simulink model "BMS_EstimateSOC_COM_Harness_SIL"  (R2022b)
settings: configuration reference "BMS_Sw_CodeGenConfig" (kept outside this file)
undefined symbols (not defined in the file): BATT, DiscIntNeverNeededParam, Ion, Lithium, Schedule
libraries: simulink x4, spsIdealSwitchLib x3, pil_lib x1, spsBatteryLib x1, spsParallelRLCBranchLib x1, spspowerguiLib x1
settings Model: DataDictionary=BMS_Arch_DD.sldd  Creator=MAAM  LastModifiedBy=MAAM
settings ConfigSetRef: SourceName=BMS_Sw_CodeGenConfig

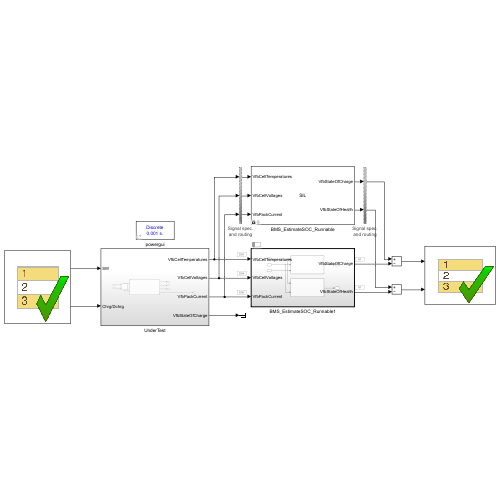
[thumbnail: Simulink's stored preview of the top-level diagram]
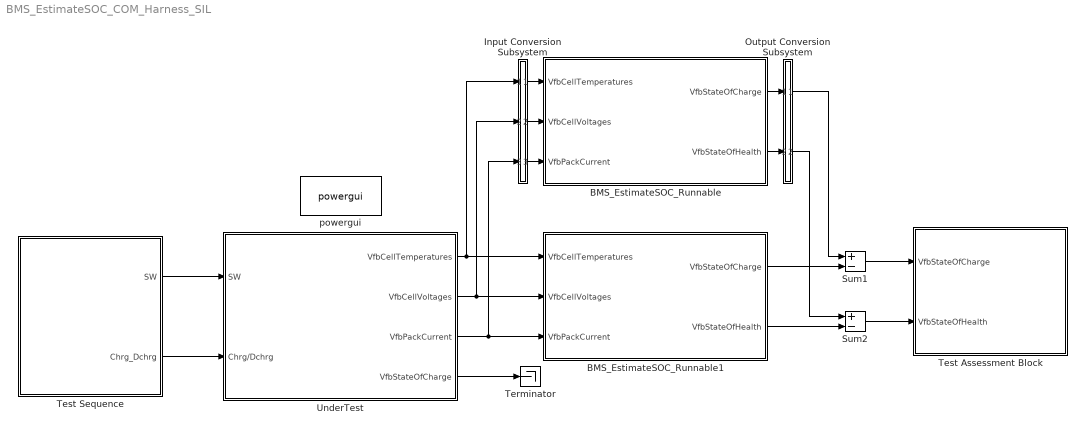
== system BMS_EstimateSOC_COM_Harness_SIL ==
  BMS_EstimateSOC_Runnable : Subsystem  Tag=__SL_testing_harness_stub_  DialogController=pil_create_dialog  LoadFcn=|
      | try
      |    if ~strcmp(rtw.pil.getPILVersion, '9.13 (R2022b)_15')
      |       set_param(gcb, 'DialogController', '');
      |       set_param(gcb, 'DialogControllerArgs', '');
      |    end
      | catch e
      |       set_param(gcb, 'DialogController', '');
      |       set_param(gcb, 'DialogControllerArgs', '');
      | end
      mask help: PIL:pil:XILBlockMaskDesc
      mask Display: disp('SIL');
  BMS_EstimateSOC_Runnable1 : Subsystem  Tag=BMS_EstimateSOC_Task  Priority=3  TreatAsAtomicUnit=on  ScheduleAs=Periodic partition  PartitionName=BMS_EstimateSOC_Task  SystemSampleTime=Schedule.BMS_EstimateSOC_Task
      settings: RTWSystemCode=Nonreusable function  RTWFcnNameOpts=Use subsystem name  FunctionInterfaceSpec=Allow arguments (Optimized)
  Input Conversion Subsystem : Subsystem  Tag=__SLT_ICS__  Description=|
      | Signal spec.
      | and routing
      settings: AttributesFormatString=%<Description>
  Output Conversion Subsystem : Subsystem  Tag=__SLT_OCS__  Description=|
      | Signal spec.
      | and routing
      settings: AttributesFormatString=%<Description>
  Sum1 : Sum  Inputs=+-
  Sum2 : Sum  Inputs=+-
  Terminator : Terminator
  Test Assessment Block : Test Sequence  Tag=__SLT_ASMT__  TreatAsAtomicUnit=on
  Test Sequence : Test Sequence  TreatAsAtomicUnit=on
  UnderTest : Subsystem
  powergui : spspowerguiLib/powergui  Priority=1  SimulationMode=Discrete  SampleTime=1e-3  frequency=60  Iterations=50  frequencyindice=0  Pbase=100e6  ErrMax=1e-4  UnitsV=kV  UnitsW=MW  buscounter=0  FunctionMessages=off  echomessages=off  EnableUseOfTLC=off  CurrentSourceSwitches=off  DisableSnubberDevices=off  DisableRonSwitches=off  DisableVfSwitches=off  DisplayEquations=off  AutomaticDiscreteSolvers=off  SolverType=Tustin/Backward Euler (TBE)  Interpol=off  ExternalGateDelay=off  methode=off  Ts=100  x0status=blocks  SPID=on  SwTol=0  HookPort=off  NonlinearTolerance=1e-4  nMaxIteration=100  ContinueOnMaxIteration=off  RestoreLinks=warning  ResistiveCurrentMeasurement=off  Frange=[0:2:500]  Ylog=off  Xlog=on  ShowGrid=off  save=off  variable=ZData  structure=0  ZoomFFT=off  StartTime=0.0  cycles=1  DisplayStyle=1  fundamental=60  FreqAxis=off  MaxFrequency=1000  frequencyindicesteady=1  RmsSteady=1  display=off
  wires:
  BMS_EstimateSOC_Runnable/1(VfbStateOfCharge) -> Output Conversion Subsystem/1(Inport_1)
  BMS_EstimateSOC_Runnable/2(VfbStateOfHealth) -> Output Conversion Subsystem/2(Inport_2)
  Input Conversion Subsystem/1(Outport_1) -> BMS_EstimateSOC_Runnable/1(VfbCellTemperatures)
  Input Conversion Subsystem/2(Outport_2) -> BMS_EstimateSOC_Runnable/2(VfbCellVoltages)
  Input Conversion Subsystem/3(Outport_3) -> BMS_EstimateSOC_Runnable/3(VfbPackCurrent)
  BMS_EstimateSOC_Runnable1/1(VfbStateOfCharge) -> Sum1/2
  BMS_EstimateSOC_Runnable1/2(VfbStateOfHealth) -> Sum2/2
  Test Sequence/1(SW) -> UnderTest/1(SW)
  Test Sequence/2(Chrg_Dchrg) -> UnderTest/2(Chrg/Dchrg)
  UnderTest/1(VfbCellTemperatures) -> Input Conversion Subsystem/1(Inport_1), BMS_EstimateSOC_Runnable1/1(VfbCellTemperatures)
  UnderTest/2(VfbCellVoltages) -> BMS_EstimateSOC_Runnable1/2(VfbCellVoltages), Input Conversion Subsystem/2(Inport_2)
  UnderTest/3(VfbPackCurrent) -> BMS_EstimateSOC_Runnable1/3(VfbPackCurrent), Input Conversion Subsystem/3(Inport_3)
  UnderTest/4(VfbStateOfCharge) -> Terminator/1
  Sum1/1 -> Test Assessment Block/1(VfbStateOfCharge)
  Sum2/1 -> Test Assessment Block/2(VfbStateOfHealth)
  Output Conversion Subsystem/2(Outport_2) -> Sum2/1
  Output Conversion Subsystem/1(Outport_1) -> Sum1/1

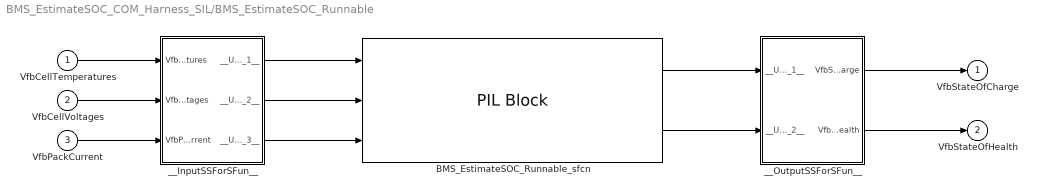
== system BMS_EstimateSOC_COM_Harness_SIL/BMS_EstimateSOC_Runnable ==
  VfbCellTemperatures : Inport  PortDimensions=BATT.Package.NumModules
  VfbCellVoltages : Inport  Port=2  PortDimensions=BATT.Package.NumModules
  VfbPackCurrent : Inport  Port=3
  BMS_EstimateSOC_Runnable_sfcn : pil_lib/PIL Block  SimulationMode=SIL  IsTopModelPIL=off  CodeDir=BMS_EstimateSOC_Runnable_ert_rtw  AnchorDir=H:\0\New MAAM\10 - MBD\Battary Management System  ConfigName=Software-in-the-Loop (SIL)  XrelIsTopModelCode=on  XrelIsReusable=off  XrelDWorkNames={}  XrelDWorkTypes={}  XrelModelArgVals={}  XrelOrderedParamNames={}
  __InputSSForSFun__ : Subsystem
  __OutputSSForSFun__ : Subsystem
  VfbStateOfCharge : Outport
  VfbStateOfHealth : Outport  Port=2
  wires:
  __OutputSSForSFun__/2(VfbStateOfHealth) -> VfbStateOfHealth/1
  __OutputSSForSFun__/1(VfbStateOfCharge) -> VfbStateOfCharge/1
  BMS_EstimateSOC_Runnable_sfcn/2 -> __OutputSSForSFun__/2(__UniqueInportName__2__)
  BMS_EstimateSOC_Runnable_sfcn/1 -> __OutputSSForSFun__/1(__UniqueInportName__1__)
  __InputSSForSFun__/3(__UniqueOutportName__3__) -> BMS_EstimateSOC_Runnable_sfcn/3
  __InputSSForSFun__/2(__UniqueOutportName__2__) -> BMS_EstimateSOC_Runnable_sfcn/2
  __InputSSForSFun__/1(__UniqueOutportName__1__) -> BMS_EstimateSOC_Runnable_sfcn/1
  VfbPackCurrent/1 -> __InputSSForSFun__/3(VfbPackCurrent)
  VfbCellVoltages/1 -> __InputSSForSFun__/2(VfbCellVoltages)
  VfbCellTemperatures/1 -> __InputSSForSFun__/1(VfbCellTemperatures)

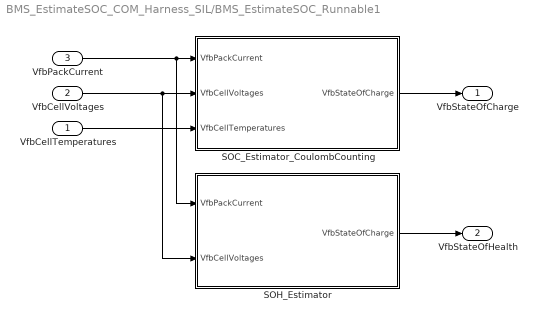
== system BMS_EstimateSOC_COM_Harness_SIL/BMS_EstimateSOC_Runnable1 ==
  VfbCellTemperatures : Inport  PortDimensions=BATT.Package.NumModules
  VfbCellVoltages : Inport  Port=2  PortDimensions=BATT.Package.NumModules
  VfbPackCurrent : Inport  Port=3
  SOC_Estimator_CoulombCounting : Subsystem  TreatAsAtomicUnit=on
      settings: RTWSystemCode=Nonreusable function  FunctionInterfaceSpec=Allow arguments (Optimized)
  SOH_Estimator : Subsystem  TreatAsAtomicUnit=on
      settings: RTWSystemCode=Nonreusable function  FunctionInterfaceSpec=Allow arguments (Optimized)
  VfbStateOfCharge : Outport
  VfbStateOfHealth : Outport  Port=2
  wires:
  SOH_Estimator/1(VfbStateOfCharge) -> VfbStateOfHealth/1
  SOC_Estimator_CoulombCounting/1(VfbStateOfCharge) -> VfbStateOfCharge/1
  VfbCellTemperatures/1 -> SOC_Estimator_CoulombCounting/3(VfbCellTemperatures)
  VfbCellVoltages/1 -> SOC_Estimator_CoulombCounting/2(VfbCellVoltages), SOH_Estimator/2(VfbCellVoltages)
  VfbPackCurrent/1 -> SOC_Estimator_CoulombCounting/1(VfbPackCurrent), SOH_Estimator/1(VfbPackCurrent)

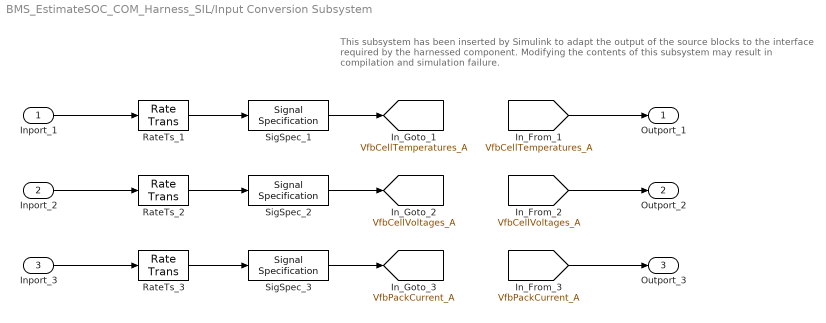
== system BMS_EstimateSOC_COM_Harness_SIL/Input Conversion Subsystem ==
  note: This subsystem has been inserted by Simulink to adapt the output of the source blocks to the interface required by the harnessed component.
      |  Modifying the contents of this subsystem may result in compilation and simulation failure.
  Inport_1 : Inport
  Inport_2 : Inport  Port=2
  Inport_3 : Inport  Port=3
  RateTs_1 : RateTransition  OutPortSampleTime=0.2
  RateTs_2 : RateTransition  OutPortSampleTime=0.2
  RateTs_3 : RateTransition  OutPortSampleTime=0.2
  SigSpec_1 : SignalSpecification  OutDataTypeStr=single  Unit=°C  Dimensions=[3]  SampleTime=0.2
  SigSpec_2 : SignalSpecification  OutDataTypeStr=single  Unit=V  Dimensions=[3]  SampleTime=0.2
  SigSpec_3 : SignalSpecification  OutDataTypeStr=single  Unit=A  Dimensions=[1]  SampleTime=0.2
  Outport_1 : Outport
  Outport_2 : Outport  Port=2
  Outport_3 : Outport  Port=3
  tag scope: VfbCellTemperatures_A=global, VfbCellVoltages_A=global, VfbPackCurrent_A=global
  wires:
  [VfbCellTemperatures_A] -> Outport_1/1
  SigSpec_1/1 -> [VfbCellTemperatures_A]
  RateTs_1/1 -> SigSpec_1/1
  Inport_1/1 -> RateTs_1/1
  [VfbCellVoltages_A] -> Outport_2/1
  SigSpec_2/1 -> [VfbCellVoltages_A]
  RateTs_2/1 -> SigSpec_2/1
  Inport_2/1 -> RateTs_2/1
  [VfbPackCurrent_A] -> Outport_3/1
  SigSpec_3/1 -> [VfbPackCurrent_A]
  RateTs_3/1 -> SigSpec_3/1
  Inport_3/1 -> RateTs_3/1

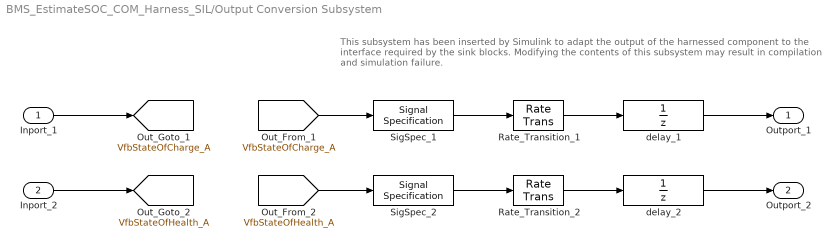
== system BMS_EstimateSOC_COM_Harness_SIL/Output Conversion Subsystem ==
  note: This subsystem has been inserted by Simulink to adapt the output of the harnessed component to the interface required by the sink blocks.
      |  Modifying the contents of this subsystem may result in compilation and simulation failure.
  Inport_1 : Inport
  Inport_2 : Inport  Port=2
  Rate_Transition_1 : RateTransition  OutPortSampleTimeOpt=Inherit
  Rate_Transition_2 : RateTransition  OutPortSampleTimeOpt=Inherit
  SigSpec_1 : SignalSpecification  OutDataTypeStr=single  Dimensions=[3]  SampleTime=0.2
  SigSpec_2 : SignalSpecification  OutDataTypeStr=single  Dimensions=[3]  SampleTime=0.2
  delay_1 : UnitDelay  SampleTime=-1
  delay_2 : UnitDelay  SampleTime=-1
  Outport_1 : Outport
  Outport_2 : Outport  Port=2
  tag scope: VfbStateOfCharge_A=global, VfbStateOfHealth_A=global
  wires:
  Inport_1/1 -> [VfbStateOfCharge_A]
  [VfbStateOfCharge_A] -> SigSpec_1/1
  SigSpec_1/1 -> Rate_Transition_1/1
  Rate_Transition_1/1 -> delay_1/1
  delay_1/1 -> Outport_1/1
  Inport_2/1 -> [VfbStateOfHealth_A]
  [VfbStateOfHealth_A] -> SigSpec_2/1
  SigSpec_2/1 -> Rate_Transition_2/1
  Rate_Transition_2/1 -> delay_2/1
  delay_2/1 -> Outport_2/1

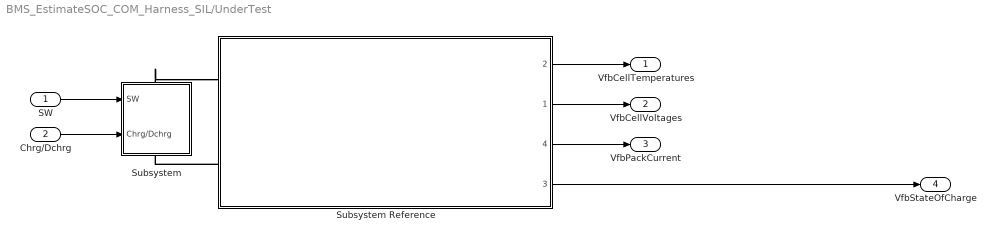
== system BMS_EstimateSOC_COM_Harness_SIL/UnderTest ==
  SW : Inport
  Chrg/Dchrg : Inport  Port=2
  Subsystem : Subsystem
      settings: PortSchema="{\"entries\":[{\"content\":{\"sides\":[{\"content\":{\"connectorIds\":[\"LConn1\"]},\"type\":\"ConnectorPlacement.EquallySpacedRectSide\",\"uuid\":\"a461fc5f-bdec-4de1-a769-19a6913359cb\"},{\"content\":{\"connectorIds\":[\"RConn1\"],\"side\":\"RIGHT\"},\"type\":\"ConnectorPlacement.EquallySpacedRectSide\",\"uuid\":\"53dfe770-afde-41f9-b1fd-6523bad3a9ef\"},{\"content\":{\"connectorIds\":[],\"side\":\"TOP\"},\"type\":\"ConnectorPlacement.EquallySpacedRectSide\",\"uuid\":\"157c2878-8b7f-49af-a18e-5ca91668c703\"},{\"content\":{\"connectorIds\":[\"In1\",\"In2\"],\"side\":\"BOTTOM\"},\"type\":\"ConnectorPlacement.EquallySpacedRectSide\",\"uuid\":\"a113e167-ab7e-4584-b97c-54a0a3809f54\"}]},\"type\":\"ConnectorPlacement.EquallySpacedConnector\",\"uuid\":\"fefc71e0-0cbe-4397-b099-f68d58411951\"}],\"packageUris\":[\"http://schema.mathworks.com/mf0/Connector/R2020b\"],\"version\":\"1.0\"}"
  Subsystem Reference : Subsystem  ReferencedSubsystem=Batter_Pack_Sim
      settings: PortSchema="{\"entries\":[{\"content\":{\"sides\":[{\"content\":{\"connectorIds\":[\"LConn1\",\"LConn2\"]},\"type\":\"ConnectorPlacement.EquallySpacedRectSide\",\"uuid\":\"5451cb71-15b5-4b08-b1e3-78543f6c5322\"},{\"content\":{\"connectorIds\":[\"Out2\",\"Out1\",\"Out4\",\"Out3\"],\"side\":\"RIGHT\"},\"type\":\"ConnectorPlacement.EquallySpacedRectSide\",\"uuid\":\"e4bd4e19-96bf-4958-bcea-cb5b9e999de9\"},{\"content\":{\"connectorIds\":[],\"side\":\"TOP\"},\"type\":\"ConnectorPlacement.EquallySpacedRectSide\",\"uuid\":\"ab10f796-18a4-45ff-a38a-380d34cf2a1b\"}]},\"type\":\"ConnectorPlacement.EquallySpacedConnector\",\"uuid\":\"eded12b9-95b7-465b-88e8-d172ae90f9f6\"}],\"packageUris\":[\"http://schema.mathworks.com/mf0/Connector/R2020b\"],\"version\":\"1.0\"}"
  VfbCellTemperatures : Outport
  VfbCellVoltages : Outport  Port=2
  VfbPackCurrent : Outport  Port=3
  VfbStateOfCharge : Outport  Port=4
  wires:
  Subsystem Reference/2 -> VfbCellTemperatures/1
  Subsystem Reference/1 -> VfbCellVoltages/1
  SW/1 -> Subsystem/1(SW)
  Subsystem Reference/3 -> VfbStateOfCharge/1
  Subsystem Reference/4 -> VfbPackCurrent/1
  Chrg/Dchrg/1 -> Subsystem/2(Chrg/Dchrg)
  connections:
  Subsystem/LConn1 -- Subsystem Reference/LConn1
  Subsystem Reference/LConn2 -- Subsystem/RConn1

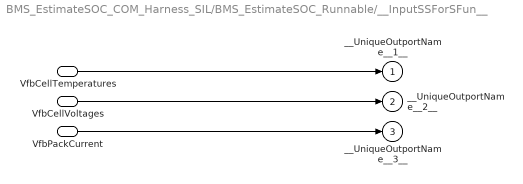
== system BMS_EstimateSOC_COM_Harness_SIL/BMS_EstimateSOC_Runnable/__InputSSForSFun__ ==
  VfbCellTemperatures : Inport  PortDimensions=BATT.Package.NumModules
  VfbCellVoltages : Inport  Port=2  PortDimensions=BATT.Package.NumModules
  VfbPackCurrent : Inport  Port=3
  __UniqueOutportName__1__ : Outport
  __UniqueOutportName__2__ : Outport  Port=2
  __UniqueOutportName__3__ : Outport  Port=3
  wires:
  VfbPackCurrent/1 -> __UniqueOutportName__3__/1
  VfbCellVoltages/1 -> __UniqueOutportName__2__/1
  VfbCellTemperatures/1 -> __UniqueOutportName__1__/1

== system BMS_EstimateSOC_COM_Harness_SIL/BMS_EstimateSOC_Runnable/__OutputSSForSFun__ ==
  __UniqueInportName__1__ : Inport
  __UniqueInportName__2__ : Inport  Port=2
  VfbStateOfCharge : Outport
  VfbStateOfHealth : Outport  Port=2
  wires:
  __UniqueInportName__2__/1 -> VfbStateOfHealth/1  "SOC"
  __UniqueInportName__1__/1 -> VfbStateOfCharge/1  "SOC"

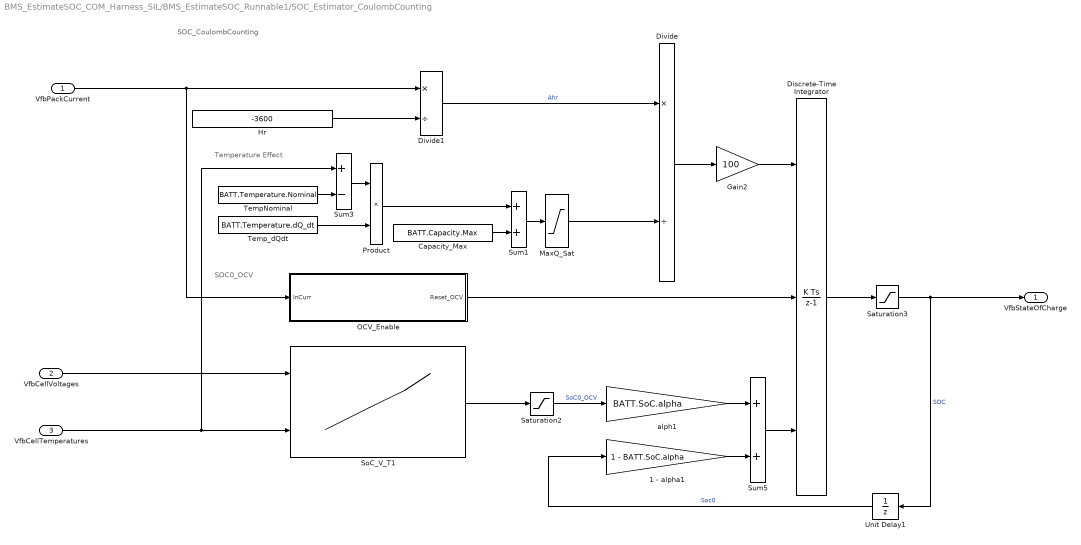
== system BMS_EstimateSOC_COM_Harness_SIL/BMS_EstimateSOC_Runnable1/SOC_Estimator_CoulombCounting ==
  note: SOC0_OCV
  note: Temperature Effect
  note: SOC_CoulombCounting
  VfbPackCurrent : Inport
  VfbCellVoltages : Inport  Port=2  PortDimensions=BATT.Package.NumModules
  VfbCellTemperatures : Inport  Port=3
  1 - alpha1 : Gain  Gain=1 - BATT.SoC.alpha
  Capacity_Max : Constant  Value=BATT.Capacity.Max
  Discrete-Time Integrator : DiscreteIntegrator  ExternalReset=rising  InitialConditionSource=external  InitialCondition=BATT.SOC.SoC0  SampleTime=-1  ICPrevOutput=DiscIntNeverNeededParam  ICPrevScaledInput=DiscIntNeverNeededParam
  Divide : Product  Inputs=*/  OutDataTypeStr=single
  Divide1 : Product  Inputs=*/
  Gain2 : Gain  Gain=100  OutDataTypeStr=single
  Hr : Constant  Value=-3600  OutDataTypeStr=single
  MaxQ_Sat : Saturate  UpperLimit=BATT.Capacity.Max  LowerLimit=0
  OCV_Enable : Subsystem
  Product : Product
  Saturation2 : Saturate  UpperLimit=BATT.SoC.max  LowerLimit=BATT.SoC.min  OutDataTypeStr=single
  Saturation3 : Saturate  UpperLimit=BATT.SoC.max  LowerLimit=BATT.SoC.min  OutDataTypeStr=single
  SoC_V_T1 : Lookup_n-D  BreakpointsForDimension1=BATT.Voltage.V_LUT  BreakpointsForDimension2=BATT.Temperature.T_LUT  Table=BATT.SoC.TableData  InternalRulePriority=Speed  RndMeth=Simplest
      settings: InputPortMap=u0,u1
  Sum1 : Sum
  Sum3 : Sum  Inputs=+-
  Sum5 : Sum
  TempNominal : Constant  Value=BATT.Temperature.Nominal
  Temp_dQdt : Constant  Value=BATT.Temperature.dQ_dt
  Unit Delay1 : UnitDelay  InitialCondition=BATT.SoC.SoC0 * ones(BATT.Package.Ns_Module, BATT.Package.NumModules)  SampleTime=-1  HasFrameUpgradeWarning=on
  alph1 : Gain  Gain=BATT.SoC.alpha
  VfbStateOfCharge : Outport
  wires:
  VfbPackCurrent/1 -> OCV_Enable/1(InCurr), Divide1/1
  VfbCellTemperatures/1 -> Sum3/1, SoC_V_T1/2
  VfbCellVoltages/1 -> SoC_V_T1/1
  Saturation3/1 -> VfbStateOfCharge/1, Unit Delay1/1  "SOC"
  TempNominal/1 -> Sum3/2
  Sum3/1 -> Product/1
  Temp_dQdt/1 -> Product/2
  Capacity_Max/1 -> Sum1/2
  Product/1 -> Sum1/1
  Sum1/1 -> MaxQ_Sat/1
  Divide1/1 -> Divide/1  "Ahr"
  Saturation2/1 -> alph1/1  "SoC0_OCV"
  Discrete-Time Integrator/1 -> Saturation3/1
  1 - alpha1/1 -> Sum5/2
  alph1/1 -> Sum5/1
  Divide/1 -> Gain2/1
  Sum5/1 -> Discrete-Time Integrator/3
  OCV_Enable/1(Reset_OCV) -> Discrete-Time Integrator/2
  Unit Delay1/1 -> 1 - alpha1/1  "Soc0"
  Gain2/1 -> Discrete-Time Integrator/1
  MaxQ_Sat/1 -> Divide/2
  Hr/1 -> Divide1/2
  SoC_V_T1/1 -> Saturation2/1

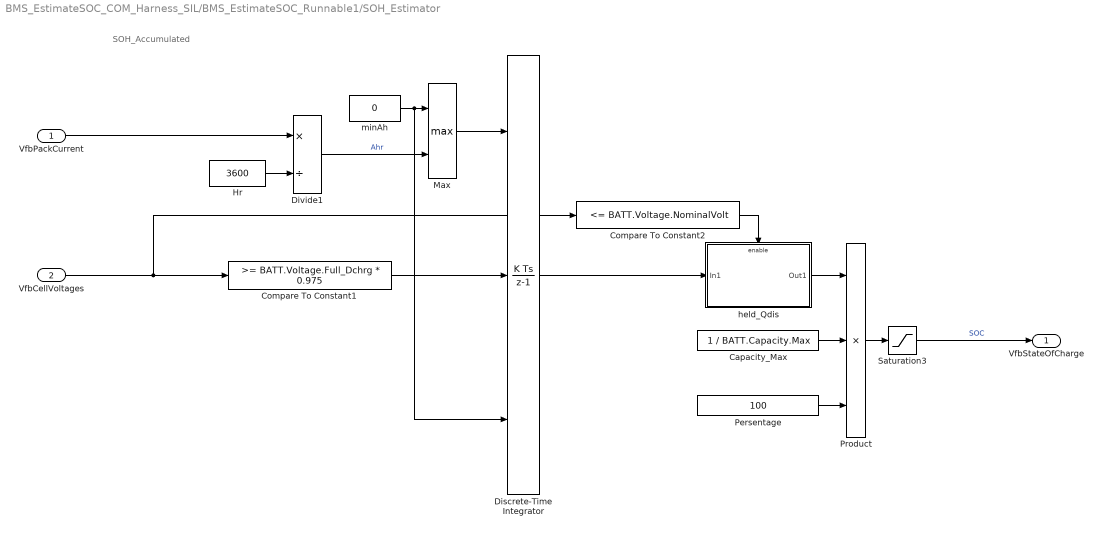
== system BMS_EstimateSOC_COM_Harness_SIL/BMS_EstimateSOC_Runnable1/SOH_Estimator ==
  note: SOH_Accumulated
  VfbPackCurrent : Inport
  VfbCellVoltages : Inport  Port=2  PortDimensions=BATT.Package.NumModules
  Capacity_Max : Constant  Value=1 / BATT.Capacity.Max
  Compare To Constant1 : simulink/Logic and Bit Operations/Compare To Constant  relop=>=  const=BATT.Voltage.Full_Dchrg * 0.975  OutDataTypeStr=boolean
  Compare To Constant2 : simulink/Logic and Bit Operations/Compare To Constant  relop=<=  const=BATT.Voltage.NominalVolt  OutDataTypeStr=boolean
  Discrete-Time Integrator : DiscreteIntegrator  ExternalReset=rising  InitialConditionSource=external  InitialCondition=BATT.SOC.SoC0  SampleTime=-1  ICPrevOutput=DiscIntNeverNeededParam  ICPrevScaledInput=DiscIntNeverNeededParam
  Divide1 : Product  Inputs=*/
  Hr : Constant  Value=3600  OutDataTypeStr=single
  Max : MinMax  Function=max  Inputs=2
  Persentage : Constant  Value=100
  Product : Product  Inputs=3
  Saturation3 : Saturate  UpperLimit=BATT.SoC.max  LowerLimit=BATT.SoC.min  OutDataTypeStr=single
  held_Qdis : Subsystem  TreatAsAtomicUnit=on
  minAh : Constant  Value=0  OutDataTypeStr=single
  VfbStateOfCharge : Outport
  wires:
  Persentage/1 -> Product/3
  Capacity_Max/1 -> Product/2
  held_Qdis/1(Out1) -> Product/1
  Compare To Constant2/1 -> held_Qdis/Enable
  Product/1 -> Saturation3/1
  Compare To Constant1/1 -> Discrete-Time Integrator/2
  Max/1 -> Discrete-Time Integrator/1
  minAh/1 -> Max/1, Discrete-Time Integrator/3
  Hr/1 -> Divide1/2
  Discrete-Time Integrator/1 -> held_Qdis/1(In1)
  Divide1/1 -> Max/2  "Ahr"
  Saturation3/1 -> VfbStateOfCharge/1  "SOC"
  VfbCellVoltages/1 -> Compare To Constant1/1, Compare To Constant2/1
  VfbPackCurrent/1 -> Divide1/1

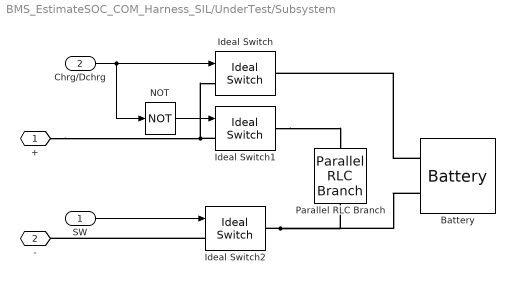
== system BMS_EstimateSOC_COM_Harness_SIL/UnderTest/Subsystem ==
  SW : Inport
  Chrg/Dchrg : Inport  Port=2
  Battery : spsBatteryLib/Battery  BatType=Lithium-Ion  ShowTempParam=off  ThermalPreset=no  ShowAgeParam=off  NomV=3*4.2  NomQ=150  SOC=100  Batt_Tr=1  PresetModel=on  MaxQ=150  MinV=9.45  FullV=14.6662  Dis_rate=65.2174  R=0.00084  Normal_OP=135.6522  expZone="[13.6129      7.36957]"  current=[6.5 13 32.5]  Units=Time  Tci=20  NomT=20  T2=-30  MaxQ2=4.8  FullV2=7.1  Normal_OP2=5.655  expZone2="[6.58           1]"  Rca=0.6  ti=2000  Dp=0  Neq0=0  Tsim=1e6  Ta1=25  Qeol=5.4*0.9  Reol=0.013333*1.2  Char_age=[2.3478, 3]  Dis_age=[2.3478, 10]  N1=1500  N2=10500  N3=1000  N4=1400  Ta2=45  N5=950
  Ideal Switch : spsIdealSwitchLib/Ideal Switch  Ron=0.001  Lon=0  IC=0  Rs=1e5  Cs=inf  Measurements=off
  Ideal Switch1 : spsIdealSwitchLib/Ideal Switch  Ron=0.001  Lon=0  IC=0  Rs=1e5  Cs=inf  Measurements=off
  Ideal Switch2 : spsIdealSwitchLib/Ideal Switch  Ron=0.001  Lon=0  IC=0  Rs=1e5  Cs=inf  Measurements=off
  NOT : Logic  Operator=NOT  IconShape=distinctive  AllPortsSameDT=off  OutDataTypeStr=boolean
  Parallel RLC Branch : spsParallelRLCBranchLib/Parallel RLC Branch  LConnTagsString=a  RConnTagsString=__new0  BranchType=R  Resistance=1  Inductance=1e-3  SetiL0=off  InitialCurrent=0  Capacitance=1e-6  Setx0=off  InitialVoltage=0  Measurements=None
  + : PMIOPort  Side=Left
  - : PMIOPort  Port=2  Side=Right
  wires:
  SW/1 -> Ideal Switch2/1
  NOT/1 -> Ideal Switch1/1
  Chrg/Dchrg/1 -> Ideal Switch/1, NOT/1
  connections:
  Ideal Switch2/LConn1 -- -/RConn1
  Ideal Switch2/RConn1 -- Parallel RLC Branch/RConn1 -- Battery/LConn2
  Ideal Switch1/RConn1 -- Parallel RLC Branch/LConn1
  +/RConn1 -- Ideal Switch/LConn1 -- Ideal Switch1/LConn1
  Battery/LConn1 -- Ideal Switch/RConn1

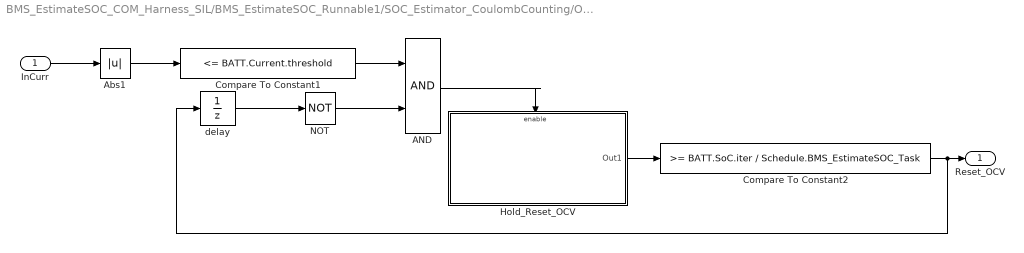
== system BMS_EstimateSOC_COM_Harness_SIL/BMS_EstimateSOC_Runnable1/SOC_Estimator_CoulombCounting/OCV_Enable ==
  InCurr : Inport
  AND : Logic  AllPortsSameDT=off  OutDataTypeStr=boolean
  Abs1 : Abs  SaturateOnIntegerOverflow=off
  Compare To Constant1 : simulink/Logic and Bit Operations/Compare To Constant  relop=<=  const=BATT.Current.threshold  OutDataTypeStr=boolean
  Compare To Constant2 : simulink/Logic and Bit Operations/Compare To Constant  relop=>=  const=BATT.SoC.iter / Schedule.BMS_EstimateSOC_Task  OutDataTypeStr=boolean
  Hold_Reset_OCV : Subsystem
  NOT : Logic  Operator=NOT  AllPortsSameDT=off  OutDataTypeStr=boolean
  delay : UnitDelay  SampleTime=-1  HasFrameUpgradeWarning=on
  Reset_OCV : Outport
  wires:
  Compare To Constant2/1 -> Reset_OCV/1, delay/1
  Abs1/1 -> Compare To Constant1/1
  AND/1 -> Hold_Reset_OCV/Enable
  delay/1 -> NOT/1
  NOT/1 -> AND/2
  Hold_Reset_OCV/1(Out1) -> Compare To Constant2/1
  Compare To Constant1/1 -> AND/1
  InCurr/1 -> Abs1/1

== system BMS_EstimateSOC_COM_Harness_SIL/BMS_EstimateSOC_Runnable1/SOH_Estimator/held_Qdis ==
  In1 : Inport
  Enable : EnablePort
  Unit Delay : UnitDelay  InitialCondition=BATT.Capacity.Max  SampleTime=-1  HasFrameUpgradeWarning=on
  Out1 : Outport
  wires:
  Unit Delay/1 -> Out1/1
  In1/1 -> Unit Delay/1

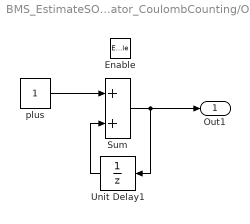
== system BMS_EstimateSOC_COM_Harness_SIL/BMS_EstimateSOC_Runnable1/SOC_Estimator_CoulombCounting/OCV_Enable/Hold_Reset_OCV ==
  Enable : EnablePort  StatesWhenEnabling=reset
  Sum : Sum
  Unit Delay1 : UnitDelay  SampleTime=-1  HasFrameUpgradeWarning=on
  plus : Constant
  Out1 : Outport  OutputWhenDisabled=reset  InitialOutput=0
  wires:
  plus/1 -> Sum/1
  Sum/1 -> Unit Delay1/1, Out1/1
  Unit Delay1/1 -> Sum/2

== stateflow chart BMS_EstimateSOC_COM_Harness_SIL/Test Assessment Block ==
  state Run
    state step_1_1
    state step_1_2
    (default) -> (junction 22)
    Run -> (junction 22)
    (junction 22) -> (junction 23) [order 1] : [t < 5
        | ]
    (junction 23) -> step_1_1 [order 1] : [~in(Run.step_1_1)]
    (junction 23) -> (junction 26) [order 2]
    (junction 31) -> (junction 32)
    (junction 32) -> step_1_2 [order 1] : [~in(Run.step_1_2)]
    (junction 32) -> (junction 35) [order 2]
    (junction 22) -> (junction 31) [order 2]
  (default) -> Run
  data: VfbStateOfCharge input single size=[3]; VfbStateOfHealth input single size=[3]

== stateflow chart BMS_EstimateSOC_COM_Harness_SIL/Test Sequence ==
  settings: updateMethod=DISCRETE  sampleTime=0.2
  state Run
    %% Initialize data outputs.
    SW = 1;
    Chrg_Dchrg = 0;
  (default) -> Run
  data: SW output single size=1; Chrg_Dchrg output single size=1
